simulink model "sixtwotwo"  (R2020a)
settings: Solver=VariableStepAuto  StartTime=0.0  StopTime=10.0  RelTol=1e-3
undefined symbols (not defined in the file or in its folder): A, B, C
settings Model: Creator=wyton  LastModifiedBy=wyton

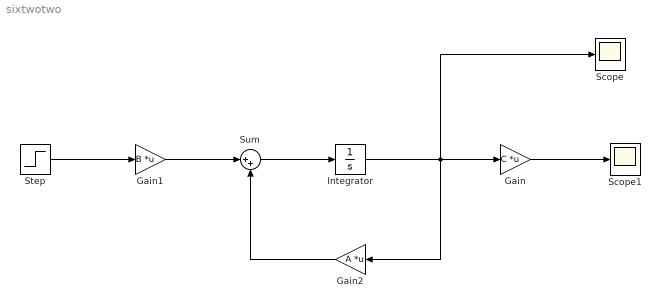
== system sixtwotwo ==
  Gain : Gain  Gain=C  Multiplication=Matrix(K*u)
  Gain1 : Gain  Gain=B  Multiplication=Matrix(K*u)
  Gain2 : Gain  Gain=A  Multiplication=Matrix(K*u)
  Integrator : Integrator
  Scope : Scope
  Scope1 : Scope
  Step : Step  Before=[0;0]  After=u  SampleTime=0
  Sum : Sum  Inputs=|++
  wires:
  Sum/1 -> Integrator/1
  Integrator/1 -> Scope/1, Gain/1, Gain2/1
  Gain/1 -> Scope1/1
  Gain2/1 -> Sum/2
  Step/1 -> Gain1/1
  Gain1/1 -> Sum/1
